simulink model "cruiseControl_v2_2018b"  (R2018b)
settings: Solver=VariableStepAuto  StartTime=0.0  StopTime=5  RelTol=1e-3
settings Model: Creator=lenovo  LastModifiedBy=lenovo

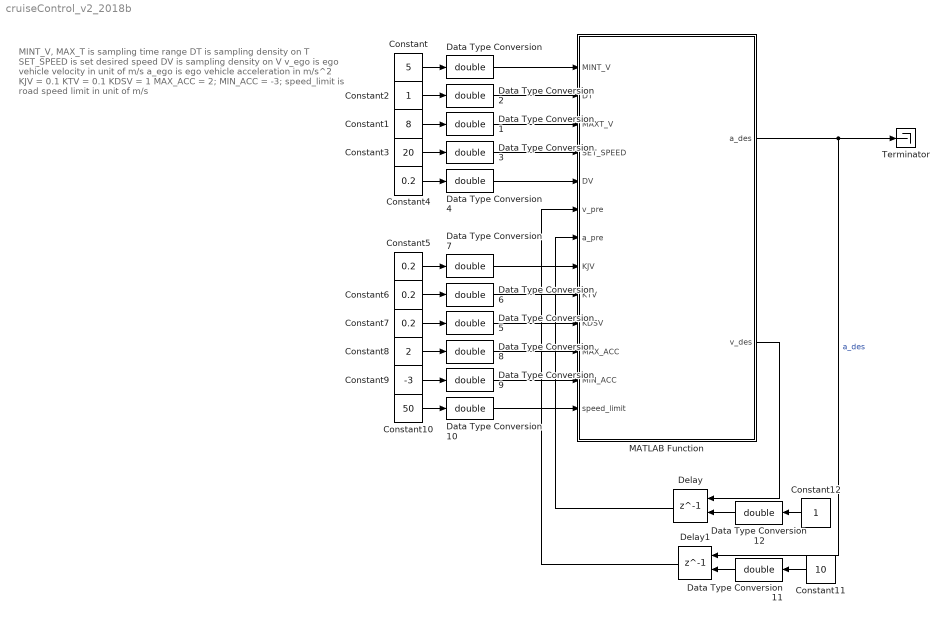
== system cruiseControl_v2_2018b ==
  note: MINT_V, MAX_T is sampling time range
      |
      | DT is sampling density on T
      |
      | SET_SPEED is set desired speed
      |
      | DV is sampling density on V
      |
      | v_ego is ego vehicle velocity in unit of m/s
      |
      | a_ego is ego vehicle acceleration in m/s^2
      |
      | KJV = 0.1
      | KTV = 0.1
      | KDSV = 1
      |
      | MAX_ACC = 2;
      | MIN_ACC = -3;
      |
      | speed_limit is road speed limit in unit of m/s
  Constant : Constant  Value=5  OutDataTypeStr=single
  Constant1 : Constant  Value=8  OutDataTypeStr=single
  Constant10 : Constant  Value=50  OutDataTypeStr=single
  Constant11 : Constant  Value=10  OutDataTypeStr=single
  Constant12 : Constant  OutDataTypeStr=single
  Constant2 : Constant  OutDataTypeStr=single
  Constant3 : Constant  Value=20  OutDataTypeStr=single
  Constant{4..7} (4 alike) : Constant  Value=0.2  OutDataTypeStr=single
  Constant8 : Constant  Value=2  OutDataTypeStr=single
  Constant9 : Constant  Value=-3  OutDataTypeStr=single
  Data Type Conversion{,1..12} (13 alike) : DataTypeConversion  OutDataTypeStr=double
  Delay : Delay  DelayLength=1  InitialConditionSource=Input port
      settings: InputPortMap=u0,p4
  Delay1 : Delay  DelayLength=1  InitialConditionSource=Input port
      settings: InputPortMap=u0,p4
  MATLAB Function : MATLAB Function  TreatAsAtomicUnit=on
  Terminator : Terminator
  wires:
  Constant/1 -> Data Type Conversion/1
  Constant1/1 -> Data Type Conversion1/1
  Data Type Conversion/1 -> MATLAB Function/1(MINT_V)
  Data Type Conversion1/1 -> MATLAB Function/3(MAXT_V)
  Constant2/1 -> Data Type Conversion2/1
  Data Type Conversion2/1 -> MATLAB Function/2(DT)
  Constant3/1 -> Data Type Conversion3/1
  Data Type Conversion3/1 -> MATLAB Function/4(SET_SPEED)
  Constant4/1 -> Data Type Conversion4/1
  Data Type Conversion4/1 -> MATLAB Function/5(DV)
  Constant7/1 -> Data Type Conversion5/1
  Constant6/1 -> Data Type Conversion6/1
  Constant5/1 -> Data Type Conversion7/1
  Data Type Conversion5/1 -> MATLAB Function/10(KDSV)
  Data Type Conversion6/1 -> MATLAB Function/9(KTV)
  Data Type Conversion7/1 -> MATLAB Function/8(KJV)
  Constant8/1 -> Data Type Conversion8/1
  Constant9/1 -> Data Type Conversion9/1
  Constant10/1 -> Data Type Conversion10/1
  Data Type Conversion8/1 -> MATLAB Function/11(MAX_ACC)
  Data Type Conversion9/1 -> MATLAB Function/12(MIN_ACC)
  Data Type Conversion10/1 -> MATLAB Function/13(speed_limit)
  MATLAB Function/1(a_des) -> Delay1/1, Terminator/1  "a_des"
  MATLAB Function/2(v_des) -> Delay/1
  Delay/1 -> MATLAB Function/7(a_pre)
  Delay1/1 -> MATLAB Function/6(v_pre)
  Constant12/1 -> Data Type Conversion12/1
  Data Type Conversion12/1 -> Delay/2
  Data Type Conversion11/1 -> Delay1/2
  Constant11/1 -> Data Type Conversion11/1

== matlab function cruiseControl_v2_2018b/MATLAB Function ==
  data: MINT_V input; a_des output; DT input; MAXT_V input; SET_SPEED input; DV input; v_pre input; a_pre input; KJV input; KTV input; KDSV input; MAX_ACC input; MIN_ACC input; speed_limit input; v_des output
function [a_des,v_des]  = fcn(MINT_V,DT,MAXT_V, SET_SPEED,DV,v_pre, a_pre,KJV, KTV, KDSV,MAX_ACC, MIN_ACC,speed_limit)


    [cost_graph] = cal_velocity_control(MINT_V,DT,MAXT_V, SET_SPEED,DV,v_pre, a_pre,KJV, KTV, KDSV); 
    [cost_optimal] = check_quantic_status(cost_graph,speed_limit, MAX_ACC, MIN_ACC); 
    [s_of_t, v_of_t,a_of_t,t_data] = combination_quantic(cost_optimal); 
    a_des = min(max(a_of_t(2),-2),3);
    v_des = min(max(v_of_t(2),0),speed_limit);
end



function [cost_graph] = cal_velocity_control(MINT_V,DT,MAXT_V, SET_SPEED,DV,v_pre, a_pre,KJV, KTV, KDSV)
    cost_graph = ones(400,11)* 500;    
    index = 1;
    delta_v = 0.1 * SET_SPEED;

    for Ti = MINT_V : DT : MAXT_V
        for Ve = SET_SPEED - 3 : DV : SET_SPEED + 3
            s0 = 0;
            v0 = v_pre;
            a0 = a_pre;
            ve = Ve;
            ae = 0;
            [a0, a1, a2, a3, a4] = quantic_polynomial(s0, ...
                v0, a0, ve, ae,Ti);
            [jerk] = cal_quantic_jerk(a3,a4,Ti);
            cost_J = mean(abs(jerk));
            cost_T = Ti;
            cost_DV = sqrt((SET_SPEED - Ve)^2);
            cost_total = KJV * cost_J + KTV * cost_T + KDSV * cost_DV;
            cost_graph(index,:) = [cost_total,Ti,Ve,cost_J,cost_T,cost_DV,...
                a0, a1, a2, a3, a4];

            index = index + 1;
        end
    end
        cost_graph = sortrows(cost_graph);
end



function [cost_optimal] = check_quantic_status(cost_graph,speed_limit, MAX_ACC, MIN_ACC,MAXT_V)
   i = 1;
    COND = 1;
    cost_optimal = zeros(1,11);
    LEN_T = 0;
    if isempty(cost_graph)
        cost_optimal=  zeros(1,11);
        fprintf("error in cost graph.");
        return;
    end
    
    valid_range = find(cost_graph(:,2) == 500);
    valid_size = valid_range(1);

    while COND == 1

        
        poly_para = cost_graph(i,7:11);
        a0 = poly_para(1); a1 = poly_para(2); a2 = poly_para(3); 
        a3 = poly_para(4); a4 = poly_para(5); 
        
        Te = cost_graph(i,2);
%         vt = [];
%         at = [];        
%         
        
%         for t = 0:0.2:Te
%             vt = [vt, calc_quantic_first_derivative(a1,a2,a3,a4,t)];
%             at = [at, calc_quantic_second_derivative(a2,a3,a4,t)];
%         end
        
        LEN_T = double(Te * 5 + 1);
        vt = zeros(200,1);
        at = zeros(200,1);
        
        for j = 1: LEN_T
            t = (j-1) * 0.2;
            vt(j) = calc_quantic_first_derivative(a1,a2,a3,a4,t);
            at(j) = calc_quantic_second_derivative(a2,a3,a4,t);
        end
        
        
        if cost_graph(i,1) == 500
            COND = 2;
        end
        
        if (max(abs(vt)) <= speed_limit && max(at) <= MAX_ACC && min(at) >= MIN_ACC)
            cost_optimal(1:11) = cost_graph(i,:);
            COND = 2;
        end
        
        i = i + 1;
        
        if i == valid_size
            COND = 2;
            POS = find(cost_graph(:,2)==MAXT_V);
            POS_first = POS(1); % find the first combination with longest T; 
            cost_optimal(1:11)  = cost_graph(POS_first,:);
        end
    end
end

function [a0, a1, a2, a3, a4] = quantic_polynomial(xs, ...
    vxs, axs, vxe, axe,T)
    
    A  =[1,0,0,0,0;0,1,0,0,0;0,0,2,0,0;...
        0,1,2*T,3*T^2,4*T^3;0,0,2,6*T,12*T^2];
    
    if det(A) == 0
        a0 = [];
        a1 = [];
        a2 = [];

        a3 = [];
        a4 = [];


        fprintf('cannot calculate quintic polynomial paras.');
        return;
    end
    
    
    b = [xs,vxs,axs,vxe,axe]';
    x = pinv(A) * b;
    
    a0 = x(1);
    a1 = x(2);
    a2 = x(3);
    a3 = x(4);
    a4 = x(5);
end

function [jerk] = cal_quantic_jerk(a3,a4,Ti)
    seg = Ti / 0.1 + 1;
    index = 1;
    jerk = zeros(1,seg);
    
    for k = 1:seg
        i  = k * 0.1;
        jerk(index) =  6* a3 + 24 * a4 * i;
        index = index + 1;
    end
end

function [s_of_t, v_of_t,a_of_t,t_data] = combination_quantic(cost_optimal)
    if isempty(cost_optimal)
        s_of_t = zeros(200,1);
        v_of_t = zeros(200,1);
        a_of_t = zeros(200,1);
        t_data = zeros(200,1);
        fprintf("error in optimal cost graph.");
        return;
    end

    Te = cost_optimal(2);
    poly_para = cost_optimal(7:11);
    a0 = poly_para(1); a1 = poly_para(2); a2 = poly_para(3); 
    a3 = poly_para(4); a4 = poly_para(5); 
    s_of_t = zeros(200,1);
    v_of_t = zeros(200,1);
    a_of_t = zeros(200,1);
    t_data = zeros(200,1);
    
    index = 1;
    seg = Te / 0.1 - 1;
    
    for i = 0 : seg
        t = i * 0.1;
        s_of_t(index) = cal_quantic_point(a0,a1,a2,a3,a4,t);
        v_of_t(index) = calc_quantic_first_derivative(a1,a2,a3,a4,t);
        a_of_t(index) = calc_quantic_second_derivative(a2,a3,a4,t);
        t_data(index) = t;
        index = index + 1;
    end
end

function [xt] = cal_quantic_point(a0,a1,a2,a3,a4,T)
    xt = a0 + a1 * T + a2 * T^2 + a3 * T^3 + a4 * T^4;
end

function [xt] =calc_quantic_first_derivative(a1,a2,a3,a4,t)
xt = a1 + 2 * a2 * t + 3 * a3 * t^2 + 4 * a4 * t^3;
end

function [xt]  = calc_quantic_second_derivative(a2,a3,a4,t)
xt = 2* a2 + 6* a3 * t + 12 * a4 * t^2;
end
